simulink library "FC_Lib"  (R2022b)
settings: Solver=VariableStepAuto  StartTime=0.0  StopTime=10.0  RelTol=1e-3
undefined symbols (not defined in the file or in its folder): DiscIntNeverNeededParam, Newton, Raphson
libraries: $bdroot x14, simulink x3, Ctrl_Lib x1
(part 2 of 2)

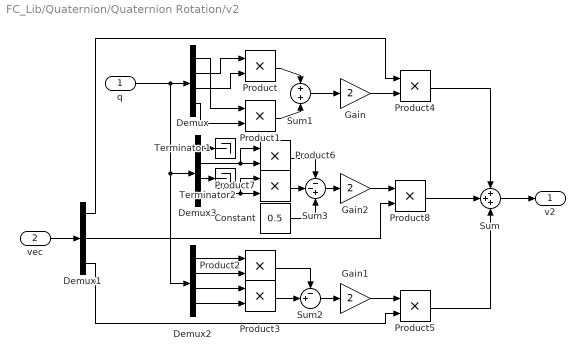
== system FC_Lib/Quaternion/Quaternion Rotation/v2 ==
  q : Inport
  vec : Inport  Port=2
  Constant : Constant  Value=0.5  OutDataTypeStr=Inherit: Inherit via back propagation
  Demux : Demux
  Demux1 : Demux  Outputs=3
  Demux2 : Demux
  Demux3 : Demux
  Gain : Gain  Gain=2  OutDataTypeStr=Inherit: Same as input
  Gain1 : Gain  Gain=2  OutDataTypeStr=Inherit: Same as input
  Gain2 : Gain  Gain=2  OutDataTypeStr=Inherit: Same as input
  Product{,1..8} (9 alike) : Product  RndMeth=Zero
  Sum : Sum  Inputs=3  AccumDataTypeStr=single
  Sum1 : Sum  Inputs=+|+
  Sum2 : Sum  Inputs=-+|
  Sum3 : Sum  Inputs=--+
  Terminator1 : Terminator
  Terminator2 : Terminator
  v2 : Outport  VectorParamsAs1DForOutWhenUnconnected=off
  wires:
  Gain1/1 -> Product5/1
  Sum2/1 -> Gain1/1
  Demux2/3 -> Product3/1
  Demux2/2 -> Product2/2
  q/1 -> Demux3/1, Demux2/1, Demux/1
  Demux2/1 -> Product2/1
  Demux2/4 -> Product3/2
  Product2/1 -> Sum2/1
  Product3/1 -> Sum2/2
  Demux3/2 -> Product6/1, Product6/2
  Sum3/1 -> Gain2/1
  Demux3/4 -> Product7/2, Product7/1
  Demux3/1 -> Terminator1/1
  Constant/1 -> Sum3/3
  Demux3/3 -> Terminator2/1
  Product6/1 -> Sum3/1
  Product7/1 -> Sum3/2
  Gain/1 -> Product4/2
  Demux/4 -> Product1/2
  Product/1 -> Sum1/1
  Sum1/1 -> Gain/1
  Demux/2 -> Product/1
  Demux/1 -> Product1/1
  Product1/1 -> Sum1/2
  Demux/3 -> Product/2
  vec/1 -> Demux1/1
  Demux1/3 -> Product5/2
  Sum/1 -> v2/1
  Product5/1 -> Sum/3
  Gain2/1 -> Product8/1
  Product4/1 -> Sum/1
  Demux1/1 -> Product4/1
  Product8/1 -> Sum/2
  Demux1/2 -> Product8/2

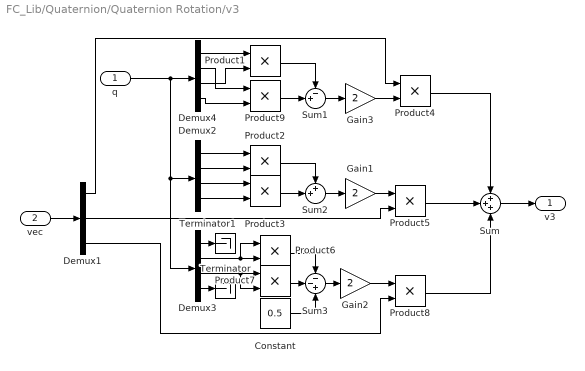
== system FC_Lib/Quaternion/Quaternion Rotation/v3 ==
  q : Inport
  vec : Inport  Port=2
  Constant : Constant  Value=0.5  OutDataTypeStr=Inherit: Inherit via back propagation
  Demux1 : Demux  Outputs=3
  Demux2 : Demux
  Demux3 : Demux
  Demux4 : Demux
  Gain1 : Gain  Gain=2  OutDataTypeStr=Inherit: Same as input
  Gain2 : Gain  Gain=2  OutDataTypeStr=Inherit: Same as input
  Gain3 : Gain  Gain=2  OutDataTypeStr=Inherit: Same as input
  Product{1..9} (9 alike) : Product  RndMeth=Zero
  Sum : Sum  Inputs=3  AccumDataTypeStr=single
  Sum1 : Sum  Inputs=-+|
  Sum2 : Sum  Inputs=++|
  Sum3 : Sum  Inputs=--+
  Terminator : Terminator
  Terminator1 : Terminator
  v3 : Outport  VectorParamsAs1DForOutWhenUnconnected=off
  wires:
  Demux3/4 -> Terminator/1
  Demux3/1 -> Terminator1/1
  Demux3/3 -> Product7/1, Product7/2
  Product6/1 -> Sum3/1
  Product7/1 -> Sum3/2
  Constant/1 -> Sum3/3
  q/1 -> Demux2/1, Demux3/1, Demux4/1
  Demux3/2 -> Product6/2, Product6/1
  Sum3/1 -> Gain2/1
  Demux2/3 -> Product3/1
  Product2/1 -> Sum2/1
  Demux2/2 -> Product2/2
  Demux2/1 -> Product2/1
  Product3/1 -> Sum2/2
  Demux2/4 -> Product3/2
  Sum2/1 -> Gain1/1
  Demux4/3 -> Product1/2
  Product9/1 -> Sum1/2
  Product1/1 -> Sum1/1
  Demux4/2 -> Product9/1
  Demux4/4 -> Product9/2
  Demux4/1 -> Product1/1
  Sum1/1 -> Gain3/1
  Demux1/3 -> Product8/2
  Product8/1 -> Sum/3
  Gain3/1 -> Product4/2
  Gain2/1 -> Product8/1
  Product4/1 -> Sum/1
  Gain1/1 -> Product5/1
  Sum/1 -> v3/1
  Demux1/2 -> Product5/2
  Product5/1 -> Sum/2
  Demux1/1 -> Product4/1
  vec/1 -> Demux1/1

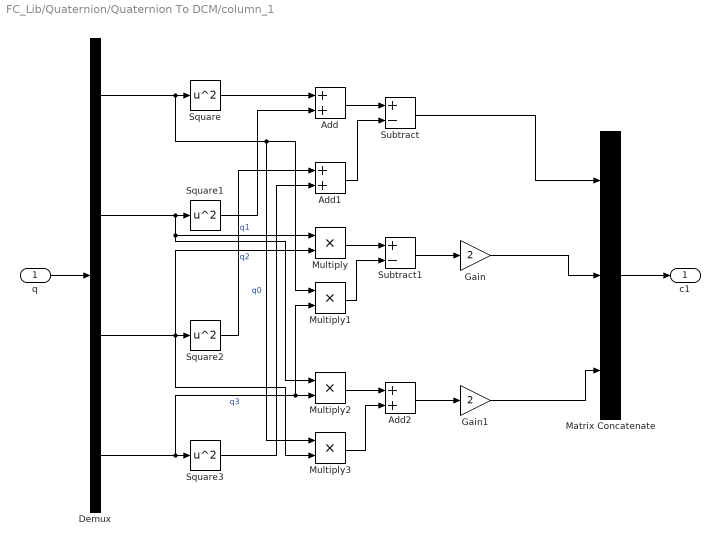
== system FC_Lib/Quaternion/Quaternion To DCM/column_1 ==
  q : Inport
  Add : Sum
  Add1 : Sum
  Add2 : Sum
  Demux : Demux
  Gain : Gain  Gain=2  OutDataTypeStr=Inherit: Same as input
  Gain1 : Gain  Gain=2  OutDataTypeStr=Inherit: Same as input
  Matrix Concatenate : Concatenate  NumInputs=3  ConcatenateDimension=2
  Multiply{,1..3} (4 alike) : Product  OutDataTypeStr=Inherit: Same as first input
  Square{,1..3} (4 alike) : Math  Operator=square  SignedPower=on
  Subtract : Sum  Inputs=+-
  Subtract1 : Sum  Inputs=+-
  c1 : Outport  VectorParamsAs1DForOutWhenUnconnected=off
  wires:
  Gain1/1 -> Matrix Concatenate/3
  Add2/1 -> Gain1/1
  Multiply3/1 -> Add2/2
  Multiply2/1 -> Add2/1
  Gain/1 -> Matrix Concatenate/2
  Subtract1/1 -> Gain/1
  Multiply1/1 -> Subtract1/2
  Multiply/1 -> Subtract1/1
  Subtract/1 -> Matrix Concatenate/1
  Add1/1 -> Subtract/2
  Add/1 -> Subtract/1
  Square3/1 -> Add1/2
  Square2/1 -> Add1/1
  Square1/1 -> Add/2
  Square/1 -> Add/1
  Demux/4 -> Square3/1, Multiply2/2, Multiply1/2  "q3"
  Demux/3 -> Multiply3/2, Square2/1, Multiply/2  "q2"
  Demux/2 -> Square1/1, Multiply2/1, Multiply/1  "q1"
  Demux/1 -> Square/1, Multiply3/1, Multiply1/1  "q0"
  Matrix Concatenate/1 -> c1/1
  q/1 -> Demux/1

== system FC_Lib/Quaternion/Quaternion To DCM/column_2 ==
  q : Inport
  Add : Sum
  Add1 : Sum
  Add3 : Sum
  Demux : Demux
  Gain : Gain  Gain=2  OutDataTypeStr=Inherit: Same as input
  Gain1 : Gain  Gain=2  OutDataTypeStr=Inherit: Same as input
  Matrix Concatenate : Concatenate  NumInputs=3  ConcatenateDimension=2
  Multiply{,1..3} (4 alike) : Product  OutDataTypeStr=Inherit: Same as first input
  Square{,1..3} (4 alike) : Math  Operator=square  SignedPower=on
  Subtract : Sum  Inputs=+-
  Subtract1 : Sum  Inputs=+-
  c2 : Outport  VectorParamsAs1DForOutWhenUnconnected=off
  wires:
  Subtract1/1 -> Gain1/1
  Multiply3/1 -> Subtract1/2
  Gain1/1 -> Matrix Concatenate/3
  Multiply2/1 -> Subtract1/1
  Subtract/1 -> Matrix Concatenate/2
  Square3/1 -> Add1/2
  Square1/1 -> Add1/1
  Square2/1 -> Add/2
  Square/1 -> Add/1
  Add1/1 -> Subtract/2
  Add/1 -> Subtract/1
  Gain/1 -> Matrix Concatenate/1
  Multiply1/1 -> Add3/2
  Multiply/1 -> Add3/1
  Add3/1 -> Gain/1
  Demux/4 -> Square3/1, Multiply2/2, Multiply1/2  "q3"
  q/1 -> Demux/1
  Demux/2 -> Multiply3/2, Square1/1, Multiply/1  "q1"
  Matrix Concatenate/1 -> c2/1
  Demux/1 -> Multiply3/1, Square/1, Multiply1/1  "q0"
  Demux/3 -> Multiply2/1, Square2/1, Multiply/2  "q2"

== system FC_Lib/Quaternion/Quaternion To DCM/column_3 ==
  q : Inport
  Add : Sum
  Add1 : Sum
  Add2 : Sum
  Demux : Demux
  Gain : Gain  Gain=2  OutDataTypeStr=Inherit: Same as input
  Gain1 : Gain  Gain=2  OutDataTypeStr=Inherit: Same as input
  Matrix Concatenate : Concatenate  NumInputs=3  ConcatenateDimension=2
  Multiply{,1..3} (4 alike) : Product  OutDataTypeStr=Inherit: Same as first input
  Square{,1..3} (4 alike) : Math  Operator=square  SignedPower=on
  Subtract : Sum  Inputs=+-
  Subtract2 : Sum  Inputs=+-
  c3 : Outport  VectorParamsAs1DForOutWhenUnconnected=off
  wires:
  Gain1/1 -> Matrix Concatenate/2
  Subtract/1 -> Matrix Concatenate/3
  Square2/1 -> Add1/2
  Square1/1 -> Add1/1
  Square3/1 -> Add/2
  Square/1 -> Add/1
  q/1 -> Demux/1
  Demux/2 -> Multiply3/2, Square1/1, Multiply/1  "q1"
  Demux/1 -> Square/1, Multiply3/1, Multiply1/1  "q0"
  Subtract2/1 -> Gain/1
  Multiply2/1 -> Add2/1
  Multiply3/1 -> Add2/2
  Matrix Concatenate/1 -> c3/1
  Multiply/1 -> Subtract2/1
  Add2/1 -> Gain1/1
  Add1/1 -> Subtract/2
  Gain/1 -> Matrix Concatenate/1
  Multiply1/1 -> Subtract2/2
  Add/1 -> Subtract/1
  Demux/3 -> Square2/1, Multiply2/1, Multiply1/2  "q2"
  Demux/4 -> Square3/1, Multiply2/2, Multiply/2  "q3"

== system FC_Lib/Transformation/LLA2FLAT/LatLon Wrap ==
  LatLon : Inport
  Constant : Constant  Value=180
  Constant1 : Constant  Value=0
  Demux : Demux  Outputs=2
  Mux : Mux  Inputs=2
  Sum : Sum  Inputs=|++
  Switch : Switch  Criteria=u2 > Threshold  SaturateOnIntegerOverflow=off  InputSameDT=off
  Weap Angle 180 : Subsystem
  Wrap Latitude : Subsystem
  LatLon_Wrap : Outport  VectorParamsAs1DForOutWhenUnconnected=off
  wires:
  LatLon/1 -> Demux/1
  Mux/1 -> LatLon_Wrap/1
  Constant/1 -> Switch/1
  Constant1/1 -> Switch/3
  Demux/1 -> Wrap Latitude/1(lat_deg)
  Wrap Latitude/2(wrap) -> Switch/2
  Wrap Latitude/1(lat_wrap) -> Mux/1
  Switch/1 -> Sum/1
  Weap Angle 180/1(angle_180) -> Mux/2
  Sum/1 -> Weap Angle 180/1(angle)
  Demux/2 -> Sum/2

== system FC_Lib/Transformation/LLA2FLAT/Rotation ==
  latlon_rad : Inport
  psio_rad : Inport  Port=2
  Demux : Demux  Outputs=2
  Multiply{1..4} (4 alike) : Product
  SinCos : Trigonometry  Operator=sincos
  Sum2 : Sum  Inputs=|++
  Sum3 : Sum  Inputs=|-+
  x_m : Outport  VectorParamsAs1DForOutWhenUnconnected=off
  y_m : Outport  Port=2  VectorParamsAs1DForOutWhenUnconnected=off
  wires:
  Sum2/1 -> x_m/1
  Multiply3/1 -> Sum3/1
  psio_rad/1 -> SinCos/1
  SinCos/2 -> Multiply1/2, Multiply4/2
  Sum3/1 -> y_m/1
  latlon_rad/1 -> Demux/1
  Multiply4/1 -> Sum3/2
  Multiply2/1 -> Sum2/2
  SinCos/1 -> Multiply2/2, Multiply3/2
  Demux/2 -> Multiply4/1, Multiply2/1
  Demux/1 -> Multiply3/1, Multiply1/1
  Multiply1/1 -> Sum2/1

== system FC_Lib/Quaternion/DCM To Quaternion/Negative Trace/Maximum Value at DCM(1,1) ==
  DCM : Inport
  Action Port : ActionPort  PropagateVarSize=During execution
  Demux : Demux  Outputs=3
      settings: DisplayOption=none
  Gain : Gain  Gain=0.5  SaturateOnIntegerOverflow=on  OutDataTypeStr=Inherit: Same as input  ParamDataTypeStr=Inherit: Same as input
  Gain1 : Gain  SaturateOnIntegerOverflow=on  OutDataTypeStr=Inherit: Same as input  ParamDataTypeStr=Inherit: Same as input
  Gain2 : Gain  SaturateOnIntegerOverflow=on  OutDataTypeStr=Inherit: Same as input  ParamDataTypeStr=Inherit: Same as input
  Gain3 : Gain  SaturateOnIntegerOverflow=on  OutDataTypeStr=Inherit: Same as input  ParamDataTypeStr=Inherit: Same as input
  Mux : Mux
  Mux1 : Mux  Inputs=3
  Product : Product  InputSameDT=on  SaturateOnIntegerOverflow=on  OutDataTypeStr=Inherit: Same as first input
  cos(phi)sin(theta)cos(psi) + sin(phi)sin(psi) -sin(theta) : Subsystem
  cos(theta)sin(phi) - (cos(phi)sin(theta)sin(psi) - sin(phi)cos(psi)) : Subsystem
  cos(theta)sin(psi) + (sin(phi)sin(theta)cos(psi) - cos(phi)sin(psi)) : Subsystem
  if s~=0; s=0.5/s : Subsystem
  sqrt : Sqrt  AlgorithmType=Newton-Raphson
  u(1) -(u(5)+u(9)) +1 : Subsystem
  qw qx qy qz : Outport  VectorParamsAs1DForOutWhenUnconnected=off
  wires:
  DCM/1 -> u(1) -(u(5)+u(9)) +1/1(DCM), cos(theta)sin(psi) + (sin(phi)sin(theta)cos(psi) - cos(phi)sin(psi))/1(DCM), cos(theta)sin(phi) - (cos(phi)sin(theta)sin(psi) - sin(phi)cos(psi))/1(DCM), cos(phi)sin(theta)cos(psi) + sin(phi)sin(psi) -sin(theta)/1(DCM)
  cos(theta)sin(psi) + (sin(phi)sin(theta)cos(psi) - cos(phi)sin(psi))/1(u(4)+u(2)) -> Mux1/1
  cos(phi)sin(theta)cos(psi) + sin(phi)sin(psi) -sin(theta)/1(u(3)+u(7)) -> Mux1/2
  cos(theta)sin(phi) - (cos(phi)sin(theta)sin(psi) - sin(phi)cos(psi))/1(u(8)-u(6)) -> Mux1/3
  Mux/1 -> qw qx qy qz/1
  u(1) -(u(5)+u(9)) +1/1(out) -> sqrt/1
  sqrt/1 -> Gain/1, if s~=0; s=0.5/s/1(s)
  Mux1/1 -> Product/2
  Demux/1 -> Gain1/1
  Demux/3 -> Gain3/1
  Demux/2 -> Gain2/1
  Gain1/1 -> Mux/3
  Gain2/1 -> Mux/4
  Gain3/1 -> Mux/1
  Product/1 -> Demux/1
  Gain/1 -> Mux/2
  if s~=0; s=0.5/s/1("s ") -> Product/1

== system FC_Lib/Quaternion/DCM To Quaternion/Negative Trace/Maximum Value at DCM(2,2) ==
  DCM : Inport
  Action Port : ActionPort  PropagateVarSize=During execution
  Demux : Demux  Outputs=3
      settings: DisplayOption=none
  Gain : Gain  Gain=0.5  SaturateOnIntegerOverflow=on  OutDataTypeStr=Inherit: Same as input  ParamDataTypeStr=Inherit: Same as input
  Gain1 : Gain  SaturateOnIntegerOverflow=on  OutDataTypeStr=Inherit: Same as input  ParamDataTypeStr=Inherit: Same as input
  Gain3 : Gain  SaturateOnIntegerOverflow=on  OutDataTypeStr=Inherit: Same as input  ParamDataTypeStr=Inherit: Same as input
  Gain4 : Gain  SaturateOnIntegerOverflow=on  OutDataTypeStr=Inherit: Same as input  ParamDataTypeStr=Inherit: Same as input
  Mux : Mux
  Mux1 : Mux  Inputs=3
  Product : Product  InputSameDT=on  SaturateOnIntegerOverflow=on  OutDataTypeStr=Inherit: Same as first input
  cos(phi)sin(theta)cos(psi) + sin(phi)sin(psi) +sin(theta) : Subsystem
  cos(theta)sin(phi) + (cos(phi)sin(theta)sin(psi) - sin(phi)cos(psi)) : Subsystem
  cos(theta)sin(psi) + (sin(phi)sin(theta)cos(psi) - cos(phi)sin(psi)) : Subsystem
  if s~=0; s=0.5/s : Subsystem
  sqrt : Sqrt  AlgorithmType=Newton-Raphson
  u(5) -(u(1)+u(9)) +1 : Subsystem
  qw qx qy qz : Outport  VectorParamsAs1DForOutWhenUnconnected=off
  wires:
  Mux1/1 -> Product/1
  DCM/1 -> u(5) -(u(1)+u(9)) +1/1(DCM), cos(phi)sin(theta)cos(psi) + sin(phi)sin(psi) +sin(theta)/1(DCM), cos(theta)sin(psi) + (sin(phi)sin(theta)cos(psi) - cos(phi)sin(psi))/1(DCM), cos(theta)sin(phi) + (cos(phi)sin(theta)sin(psi) - sin(phi)cos(psi))/1(DCM)
  cos(theta)sin(psi) + (sin(phi)sin(theta)cos(psi) - cos(phi)sin(psi))/1(u(4)+u(2)) -> Mux1/1
  cos(theta)sin(phi) + (cos(phi)sin(theta)sin(psi) - sin(phi)cos(psi))/1(u(8)+u(6)) -> Mux1/2
  cos(phi)sin(theta)cos(psi) + sin(phi)sin(psi) +sin(theta)/1(u(3)-u(7)) -> Mux1/3
  Mux/1 -> qw qx qy qz/1
  u(5) -(u(1)+u(9)) +1/1(out) -> sqrt/1
  Gain/1 -> Mux/3
  Product/1 -> Demux/1
  Demux/1 -> Gain1/1
  Demux/2 -> Gain3/1
  Demux/3 -> Gain4/1
  Gain1/1 -> Mux/2
  Gain3/1 -> Mux/4
  Gain4/1 -> Mux/1
  if s~=0; s=0.5/s/1("s ") -> Product/2
  sqrt/1 -> if s~=0; s=0.5/s/1(s), Gain/1

== system FC_Lib/Quaternion/DCM To Quaternion/Negative Trace/Maximum Value at DCM(3,3) ==
  DCM : Inport
  Action Port : ActionPort  PropagateVarSize=During execution
  Demux : Demux  Outputs=3
      settings: DisplayOption=none
  Gain : Gain  Gain=0.5  SaturateOnIntegerOverflow=on  OutDataTypeStr=Inherit: Same as input  ParamDataTypeStr=Inherit: Same as input
  Gain1 : Gain  SaturateOnIntegerOverflow=on  OutDataTypeStr=Inherit: Same as input  ParamDataTypeStr=Inherit: Same as input
  Gain2 : Gain  SaturateOnIntegerOverflow=on  OutDataTypeStr=Inherit: Same as input  ParamDataTypeStr=Inherit: Same as input
  Gain3 : Gain  SaturateOnIntegerOverflow=on  OutDataTypeStr=Inherit: Same as input  ParamDataTypeStr=Inherit: Same as input
  Mux : Mux
  Mux1 : Mux  Inputs=3
  Product : Product  InputSameDT=on  SaturateOnIntegerOverflow=on  OutDataTypeStr=Inherit: Same as first input
  cos(phi)sin(theta)cos(psi) + sin(phi)sin(psi) -sin(theta) : Subsystem
  cos(theta)sin(phi) + (cos(phi)sin(theta)sin(psi) - sin(phi)cos(psi)) : Subsystem
  cos(theta)sin(psi) - (sin(phi)sin(theta)cos(psi) - cos(phi)sin(psi)) : Subsystem
  if s~=0; s=0.5/s : Subsystem
  sqrt : Sqrt  AlgorithmType=Newton-Raphson
  u(9) -(u(1)+u(5)) +1 : Subsystem
  qw qx qy qz : Outport  VectorParamsAs1DForOutWhenUnconnected=off
  wires:
  Mux1/1 -> Product/1
  DCM/1 -> u(9) -(u(1)+u(5)) +1/1(DCM), cos(theta)sin(psi) - (sin(phi)sin(theta)cos(psi) - cos(phi)sin(psi))/1(DCM), cos(theta)sin(phi) + (cos(phi)sin(theta)sin(psi) - sin(phi)cos(psi))/1(DCM), cos(phi)sin(theta)cos(psi) + sin(phi)sin(psi) -sin(theta)/1(DCM)
  cos(phi)sin(theta)cos(psi) + sin(phi)sin(psi) -sin(theta)/1(u(3)+u(7)) -> Mux1/1
  cos(theta)sin(phi) + (cos(phi)sin(theta)sin(psi) - sin(phi)cos(psi))/1(u(8)+u(6)) -> Mux1/2
  cos(theta)sin(psi) - (sin(phi)sin(theta)cos(psi) - cos(phi)sin(psi))/1(u(4)-u(2)) -> Mux1/3
  Mux/1 -> qw qx qy qz/1
  u(9) -(u(1)+u(5)) +1/1(out) -> sqrt/1
  sqrt/1 -> Gain/1, if s~=0; s=0.5/s/1(s)
  Product/1 -> Demux/1
  Demux/1 -> Gain1/1
  Demux/3 -> Gain3/1
  Demux/2 -> Gain2/1
  Gain/1 -> Mux/4
  Gain1/1 -> Mux/2
  Gain2/1 -> Mux/3
  Gain3/1 -> Mux/1
  if s~=0; s=0.5/s/1("s ") -> Product/2

== system FC_Lib/Quaternion/DCM To Quaternion/Negative Trace/diag(DCM) ==
  DCM : Inport
  Demux : Demux  Outputs=3
  Selector : Selector  InputPortWidth=9  IndexOptions=Index vector (dialog)  Indices=[1 5 9]  OutputSizes=1
  u(1) : Outport  VectorParamsAs1DForOutWhenUnconnected=off
  u(5) : Outport  Port=2  VectorParamsAs1DForOutWhenUnconnected=off
  u(9) : Outport  Port=3  VectorParamsAs1DForOutWhenUnconnected=off
  wires:
  DCM/1 -> Selector/1
  Demux/1 -> u(1)/1
  Demux/2 -> u(5)/1
  Demux/3 -> u(9)/1
  Selector/1 -> Demux/1

== system FC_Lib/Quaternion/DCM To Quaternion/Positive Trace/cos(phi)sin(theta)cos(psi) + sin(phi)sin(psi) +sin(theta) ==
  DCM : Inport
  Add : Sum  Inputs=+-|
  Demux : Demux  Outputs=2
  Selector : Selector  InputPortWidth=9  IndexOptions=Index vector (dialog)  Indices=[3 7]  OutputSizes=1
  u(3)-u(7) : Outport  VectorParamsAs1DForOutWhenUnconnected=off
  wires:
  DCM/1 -> Selector/1
  Add/1 -> u(3)-u(7)/1
  Selector/1 -> Demux/1
  Demux/2 -> Add/2
  Demux/1 -> Add/1

== system FC_Lib/Quaternion/DCM To Quaternion/Positive Trace/cos(theta)sin(phi) - (cos(phi)sin(theta)sin(psi) - sin(phi)cos(psi)) ==
  DCM : Inport
  Add : Sum  Inputs=|-+
  Demux : Demux  Outputs=2
  Selector : Selector  InputPortWidth=9  IndexOptions=Index vector (dialog)  Indices=[6 8]  OutputSizes=1
  u(8)-u(6) : Outport  VectorParamsAs1DForOutWhenUnconnected=off
  wires:
  Add/1 -> u(8)-u(6)/1
  DCM/1 -> Selector/1
  Demux/1 -> Add/1
  Demux/2 -> Add/2
  Selector/1 -> Demux/1

== system FC_Lib/Quaternion/DCM To Quaternion/Positive Trace/cos(theta)sin(psi) - (sin(phi)sin(theta)cos(psi) - cos(phi)sin(psi)) ==
  DCM : Inport
  Add : Sum  Inputs=|-+
  Demux : Demux  Outputs=2
  Selector : Selector  InputPortWidth=9  IndexOptions=Index vector (dialog)  Indices=[2 4]  OutputSizes=1
  u(4)-u(2) : Outport  VectorParamsAs1DForOutWhenUnconnected=off
  wires:
  Add/1 -> u(4)-u(2)/1
  DCM/1 -> Selector/1
  Selector/1 -> Demux/1
  Demux/1 -> Add/1
  Demux/2 -> Add/2

== system FC_Lib/Transformation/LLA2FLAT/LatLon Wrap/Weap Angle 180 ==
  angle : Inport
  Abs1 : Abs  SaturateOnIntegerOverflow=off
  Bias2 : Bias  Bias=180  SaturateOnIntegerOverflow=off
  Bias3 : Bias  Bias=-180  SaturateOnIntegerOverflow=off
  Compare To Constant1 : simulink/Logic and Bit Operations/Compare To Constant  relop=>  const=180  OutDataTypeStr=boolean
  Constant : Constant  Value=360
  Math Function : Math  Operator=mod  SignedPower=on
  Switch1 : Switch  Criteria=u2 ~= 0  SaturateOnIntegerOverflow=off  InputSameDT=off
  angle_180 : Outport  VectorParamsAs1DForOutWhenUnconnected=off
  wires:
  Abs1/1 -> Compare To Constant1/1
  Compare To Constant1/1 -> Switch1/2
  angle/1 -> Switch1/3, Bias2/1, Abs1/1
  Bias2/1 -> Math Function/1
  Constant/1 -> Math Function/2
  Math Function/1 -> Bias3/1
  Bias3/1 -> Switch1/1
  Switch1/1 -> angle_180/1

== system FC_Lib/Transformation/LLA2FLAT/LatLon Wrap/Wrap Latitude ==
  lat_deg : Inport
  Abs : Abs  SaturateOnIntegerOverflow=off
  Bias2 : Bias  Bias=-90  SaturateOnIntegerOverflow=off
  Bias3 : Bias  Bias=90  SaturateOnIntegerOverflow=off
  Compare To Constant1 : simulink/Logic and Bit Operations/Compare To Constant  relop=>  const=90  OutDataTypeStr=boolean
  Gain1 : Gain  Gain=-1
  Multiply : Product
  Sign : Signum
  Switch1 : Switch  Criteria=u2 ~= 0  SaturateOnIntegerOverflow=off  InputSameDT=off
  Weap Angle 180 : Subsystem
  lat_wrap : Outport  VectorParamsAs1DForOutWhenUnconnected=off
  wrap : Outport  Port=2  VectorParamsAs1DForOutWhenUnconnected=off
  wires:
  lat_deg/1 -> Switch1/3, Weap Angle 180/1(angle), Abs/1
  Weap Angle 180/1(angle_180) -> Sign/1
  Sign/1 -> Multiply/1
  Bias2/1 -> Gain1/1
  Gain1/1 -> Bias3/1
  Bias3/1 -> Multiply/2
  Abs/1 -> Bias2/1, Compare To Constant1/1
  Compare To Constant1/1 -> wrap/1, Switch1/2
  Multiply/1 -> Switch1/1
  Switch1/1 -> lat_wrap/1

== system FC_Lib/Quaternion/DCM To Quaternion/Negative Trace/Maximum Value at DCM(1,1)/cos(phi)sin(theta)cos(psi) + sin(phi)sin(psi) -sin(theta) ==
  DCM : Inport
  Add : Sum  Inputs=++|
  Demux : Demux  Outputs=2
  Selector : Selector  InputPortWidth=9  IndexOptions=Index vector (dialog)  Indices=[3 7]  OutputSizes=1
  u(3)+u(7) : Outport  VectorParamsAs1DForOutWhenUnconnected=off
  wires:
  DCM/1 -> Selector/1
  Add/1 -> u(3)+u(7)/1
  Demux/2 -> Add/2
  Demux/1 -> Add/1
  Selector/1 -> Demux/1

== system FC_Lib/Quaternion/DCM To Quaternion/Negative Trace/Maximum Value at DCM(1,1)/cos(theta)sin(phi) - (cos(phi)sin(theta)sin(psi) - sin(phi)cos(psi)) ==
  DCM : Inport
  Add : Sum  Inputs=|-+
  Demux : Demux  Outputs=2
  Selector : Selector  InputPortWidth=9  IndexOptions=Index vector (dialog)  Indices=[6 8]  OutputSizes=1
  u(8)-u(6) : Outport  VectorParamsAs1DForOutWhenUnconnected=off
  wires:
  DCM/1 -> Selector/1
  Add/1 -> u(8)-u(6)/1
  Selector/1 -> Demux/1
  Demux/1 -> Add/1
  Demux/2 -> Add/2

== system FC_Lib/Quaternion/DCM To Quaternion/Negative Trace/Maximum Value at DCM(1,1)/cos(theta)sin(psi) + (sin(phi)sin(theta)cos(psi) - cos(phi)sin(psi)) ==
  DCM : Inport
  Add : Sum  Inputs=|++
  Demux : Demux  Outputs=2
  Selector : Selector  InputPortWidth=9  IndexOptions=Index vector (dialog)  Indices=[2 4]  OutputSizes=1
  u(4)+u(2) : Outport  VectorParamsAs1DForOutWhenUnconnected=off
  wires:
  Add/1 -> u(4)+u(2)/1
  DCM/1 -> Selector/1
  Selector/1 -> Demux/1
  Demux/1 -> Add/1
  Demux/2 -> Add/2

== system FC_Lib/Quaternion/DCM To Quaternion/Negative Trace/Maximum Value at DCM(1,1)/if s~=0; s=0.5//s ==
  s : Inport
  Constant1 : Constant  Value=0.5  OutDataTypeStr=Inherit: Inherit via back propagation
  Constant2 : Constant  Value=[0 1]  OutDataTypeStr=Inherit: Inherit via back propagation
  Demux : Demux  Outputs=2
  Mux : Mux  Inputs=2
  Product : Product  Inputs=*/  RndMeth=Zero
  Switch : Switch  Criteria=u2 ~= 0
  "s " : Outport  VectorParamsAs1DForOutWhenUnconnected=off
  wires:
  Demux/1 -> Product/1
  Demux/2 -> Product/2
  Constant1/1 -> Mux/1
  Mux/1 -> Switch/1
  s/1 -> Switch/2, Mux/2
  Switch/1 -> Demux/1
  Constant2/1 -> Switch/3
  Product/1 -> "s "/1

== system FC_Lib/Quaternion/DCM To Quaternion/Negative Trace/Maximum Value at DCM(1,1)/u(1) -(u(5)+u(9)) +1 ==
  DCM : Inport
  Add : Sum  Inputs=+--+
  Constant : Constant  OutDataTypeStr=Inherit: Inherit via back propagation
  Demux : Demux  Outputs=3
  Selector : Selector  InputPortWidth=9  IndexOptions=Index vector (dialog)  Indices=[1 5 9]  OutputSizes=1
  out : Outport  VectorParamsAs1DForOutWhenUnconnected=off
  wires:
  Add/1 -> out/1
  DCM/1 -> Selector/1
  Constant/1 -> Add/4
  Selector/1 -> Demux/1
  Demux/2 -> Add/2
  Demux/1 -> Add/1
  Demux/3 -> Add/3

== system FC_Lib/Quaternion/DCM To Quaternion/Negative Trace/Maximum Value at DCM(2,2)/cos(phi)sin(theta)cos(psi) + sin(phi)sin(psi) +sin(theta) ==
  DCM : Inport
  Add : Sum  Inputs=+-|
  Demux : Demux  Outputs=2
  Selector : Selector  InputPortWidth=9  IndexOptions=Index vector (dialog)  Indices=[3 7]  OutputSizes=1
  u(3)-u(7) : Outport  VectorParamsAs1DForOutWhenUnconnected=off
  wires:
  Add/1 -> u(3)-u(7)/1
  Demux/2 -> Add/2
  DCM/1 -> Selector/1
  Demux/1 -> Add/1
  Selector/1 -> Demux/1

== system FC_Lib/Quaternion/DCM To Quaternion/Negative Trace/Maximum Value at DCM(2,2)/cos(theta)sin(phi) + (cos(phi)sin(theta)sin(psi) - sin(phi)cos(psi)) ==
  DCM : Inport
  Add : Sum  Inputs=|++
  Demux : Demux  Outputs=2
  Selector : Selector  InputPortWidth=9  IndexOptions=Index vector (dialog)  Indices=[6 8]  OutputSizes=1
  u(8)+u(6) : Outport  VectorParamsAs1DForOutWhenUnconnected=off
  wires:
  Add/1 -> u(8)+u(6)/1
  DCM/1 -> Selector/1
  Selector/1 -> Demux/1
  Demux/1 -> Add/1
  Demux/2 -> Add/2

== system FC_Lib/Quaternion/DCM To Quaternion/Negative Trace/Maximum Value at DCM(2,2)/cos(theta)sin(psi) + (sin(phi)sin(theta)cos(psi) - cos(phi)sin(psi)) ==
  DCM : Inport
  Add : Sum  Inputs=|++
  Demux : Demux  Outputs=2
  Selector : Selector  InputPortWidth=9  IndexOptions=Index vector (dialog)  Indices=[2 4]  OutputSizes=1
  u(4)+u(2) : Outport  VectorParamsAs1DForOutWhenUnconnected=off
  wires:
  DCM/1 -> Selector/1
  Add/1 -> u(4)+u(2)/1
  Selector/1 -> Demux/1
  Demux/1 -> Add/1
  Demux/2 -> Add/2

== system FC_Lib/Quaternion/DCM To Quaternion/Negative Trace/Maximum Value at DCM(2,2)/if s~=0; s=0.5//s ==
  s : Inport
  Constant1 : Constant  Value=0.5  OutDataTypeStr=Inherit: Inherit via back propagation
  Constant2 : Constant  Value=[0 1]  OutDataTypeStr=Inherit: Inherit via back propagation
  Demux : Demux  Outputs=2
  Mux : Mux  Inputs=2
  Product : Product  Inputs=*/  RndMeth=Zero
  Switch : Switch  Criteria=u2 ~= 0
  "s " : Outport  VectorParamsAs1DForOutWhenUnconnected=off
  wires:
  Product/1 -> "s "/1
  Constant2/1 -> Switch/3
  Switch/1 -> Demux/1
  s/1 -> Mux/2, Switch/2
  Mux/1 -> Switch/1
  Constant1/1 -> Mux/1
  Demux/2 -> Product/2
  Demux/1 -> Product/1

== system FC_Lib/Quaternion/DCM To Quaternion/Negative Trace/Maximum Value at DCM(2,2)/u(5) -(u(1)+u(9)) +1 ==
  DCM : Inport
  Add : Sum  Inputs=-+-+
  Constant : Constant  OutDataTypeStr=Inherit: Inherit via back propagation
  Demux : Demux  Outputs=3
  Selector : Selector  InputPortWidth=9  IndexOptions=Index vector (dialog)  Indices=[1 5 9]  OutputSizes=1
  out : Outport  VectorParamsAs1DForOutWhenUnconnected=off
  wires:
  Constant/1 -> Add/4
  DCM/1 -> Selector/1
  Add/1 -> out/1
  Selector/1 -> Demux/1
  Demux/2 -> Add/2
  Demux/1 -> Add/1
  Demux/3 -> Add/3

== system FC_Lib/Quaternion/DCM To Quaternion/Negative Trace/Maximum Value at DCM(3,3)/cos(phi)sin(theta)cos(psi) + sin(phi)sin(psi) -sin(theta) ==
  DCM : Inport
  Add : Sum  Inputs=++|
  Demux : Demux  Outputs=2
  Selector : Selector  InputPortWidth=9  IndexOptions=Index vector (dialog)  Indices=[3 7]  OutputSizes=1
  u(3)+u(7) : Outport  VectorParamsAs1DForOutWhenUnconnected=off
  wires:
  Add/1 -> u(3)+u(7)/1
  DCM/1 -> Selector/1
  Demux/2 -> Add/2
  Demux/1 -> Add/1
  Selector/1 -> Demux/1

== system FC_Lib/Quaternion/DCM To Quaternion/Negative Trace/Maximum Value at DCM(3,3)/cos(theta)sin(phi) + (cos(phi)sin(theta)sin(psi) - sin(phi)cos(psi)) ==
  DCM : Inport
  Add : Sum  Inputs=|++
  Demux : Demux  Outputs=2
  Selector : Selector  InputPortWidth=9  IndexOptions=Index vector (dialog)  Indices=[6 8]  OutputSizes=1
  u(8)+u(6) : Outport  VectorParamsAs1DForOutWhenUnconnected=off
  wires:
  DCM/1 -> Selector/1
  Add/1 -> u(8)+u(6)/1
  Selector/1 -> Demux/1
  Demux/1 -> Add/1
  Demux/2 -> Add/2

== system FC_Lib/Quaternion/DCM To Quaternion/Negative Trace/Maximum Value at DCM(3,3)/cos(theta)sin(psi) - (sin(phi)sin(theta)cos(psi) - cos(phi)sin(psi)) ==
  DCM : Inport
  Add : Sum  Inputs=|-+
  Demux : Demux  Outputs=2
  Selector : Selector  InputPortWidth=9  IndexOptions=Index vector (dialog)  Indices=[2 4]  OutputSizes=1
  u(4)-u(2) : Outport  VectorParamsAs1DForOutWhenUnconnected=off
  wires:
  DCM/1 -> Selector/1
  Add/1 -> u(4)-u(2)/1
  Selector/1 -> Demux/1
  Demux/1 -> Add/1
  Demux/2 -> Add/2

== system FC_Lib/Quaternion/DCM To Quaternion/Negative Trace/Maximum Value at DCM(3,3)/if s~=0; s=0.5//s ==
  s : Inport
  Constant1 : Constant  Value=0.5  OutDataTypeStr=Inherit: Inherit via back propagation
  Constant2 : Constant  Value=[0 1]  OutDataTypeStr=Inherit: Inherit via back propagation
  Demux : Demux  Outputs=2
  Mux : Mux  Inputs=2
  Product : Product  Inputs=*/  RndMeth=Zero
  Switch : Switch  Criteria=u2 ~= 0
  "s " : Outport  VectorParamsAs1DForOutWhenUnconnected=off
  wires:
  Demux/1 -> Product/1
  Demux/2 -> Product/2
  Constant1/1 -> Mux/1
  Mux/1 -> Switch/1
  s/1 -> Switch/2, Mux/2
  Switch/1 -> Demux/1
  Constant2/1 -> Switch/3
  Product/1 -> "s "/1

== system FC_Lib/Quaternion/DCM To Quaternion/Negative Trace/Maximum Value at DCM(3,3)/u(9) -(u(1)+u(5)) +1 ==
  DCM : Inport
  Add : Sum  Inputs=--++
  Constant : Constant  OutDataTypeStr=Inherit: Inherit via back propagation
  Demux : Demux  Outputs=3
  Selector : Selector  InputPortWidth=9  IndexOptions=Index vector (dialog)  Indices=[1 5 9]  OutputSizes=1
  out : Outport  VectorParamsAs1DForOutWhenUnconnected=off
  wires:
  Constant/1 -> Add/4
  DCM/1 -> Selector/1
  Add/1 -> out/1
  Selector/1 -> Demux/1
  Demux/2 -> Add/2
  Demux/1 -> Add/1
  Demux/3 -> Add/3

== system FC_Lib/Transformation/LLA2FLAT/LatLon Wrap/Wrap Latitude/Weap Angle 180 ==
  angle : Inport
  Abs1 : Abs  SaturateOnIntegerOverflow=off
  Bias2 : Bias  Bias=180  SaturateOnIntegerOverflow=off
  Bias3 : Bias  Bias=-180  SaturateOnIntegerOverflow=off
  Compare To Constant1 : simulink/Logic and Bit Operations/Compare To Constant  relop=>  const=180  OutDataTypeStr=boolean
  Constant : Constant  Value=360
  Math Function : Math  Operator=mod  SignedPower=on
  Switch1 : Switch  Criteria=u2 ~= 0  SaturateOnIntegerOverflow=off  InputSameDT=off
  angle_180 : Outport  VectorParamsAs1DForOutWhenUnconnected=off
  wires:
  Abs1/1 -> Compare To Constant1/1
  Compare To Constant1/1 -> Switch1/2
  angle/1 -> Switch1/3, Bias2/1, Abs1/1
  Bias2/1 -> Math Function/1
  Constant/1 -> Math Function/2
  Math Function/1 -> Bias3/1
  Bias3/1 -> Switch1/1
  Switch1/1 -> angle_180/1

== matlab function FC_Lib/Fromation/Consensus Controller ==
  data: psi input; delta_xyz input; ux_cmd output; delta_v input; uy_cmd output; adj_matrix parameter; uav_id parameter; rel_x parameter; rel_y parameter; uz_cmd output; rel_z parameter; x_limit parameter; y_limit parameter; z_limit parameter
function [ux_cmd, uy_cmd, uz_cmd] = fcn(psi, delta_xyz, delta_v, adj_matrix, uav_id, rel_x, rel_y, rel_z, x_limit, y_limit, z_limit)
num = size(adj_matrix, 1);
ux_cmd = zeros(1, "like", delta_xyz(1,1));
uy_cmd = ux_cmd;
uz_cmd = ux_cmd;
dcm = [cos(psi) sin(psi);-sin(psi) cos(psi)];
for j = 1:num
    new_delta_xy = dcm * [delta_xyz(j,1) ;delta_xyz(j,2)];
    new_delta_vxy = dcm * [delta_v(j,1) ;delta_v(j,2)];
    ux_cmd = ux_cmd - adj_matrix(uav_id, j) * ((new_delta_xy(1) - rel_x(uav_id, j)) + 1 * new_delta_vxy(1));
    uy_cmd = uy_cmd - adj_matrix(uav_id, j) * ((new_delta_xy(2) - rel_y(uav_id, j)) + 1 * new_delta_vxy(2));
    uz_cmd = uz_cmd - adj_matrix(uav_id, j) * ((delta_xyz(j,3) - rel_z(uav_id, j)) + 0 * (delta_v(j, 3)));
end
ux_cmd = max(min(ux_cmd, x_limit), -x_limit);
uy_cmd = max(min(uy_cmd, y_limit), -y_limit);
uz_cmd = max(min(uz_cmd, z_limit), -z_limit);

end
